simulink model "udp_signal"  (R2025b)
settings: Solver=VariableStepAuto  StartTime=0.0  StopTime=3600  RelTol=1e-3
undefined symbols (not defined in the file or in its folder): f
libraries: instrumentlib x2
settings Model: Creator=mateu  LastModifiedBy=mateu

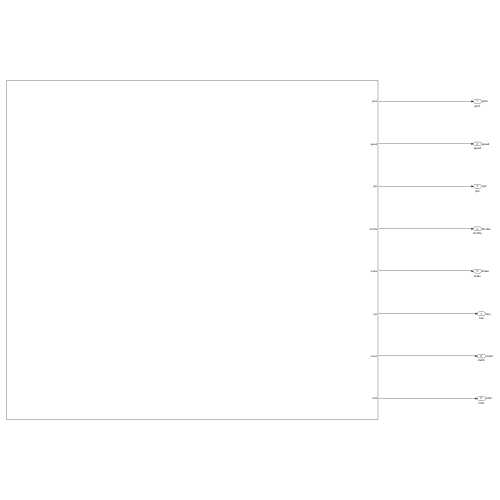
[thumbnail: Simulink's stored preview of the top-level diagram]
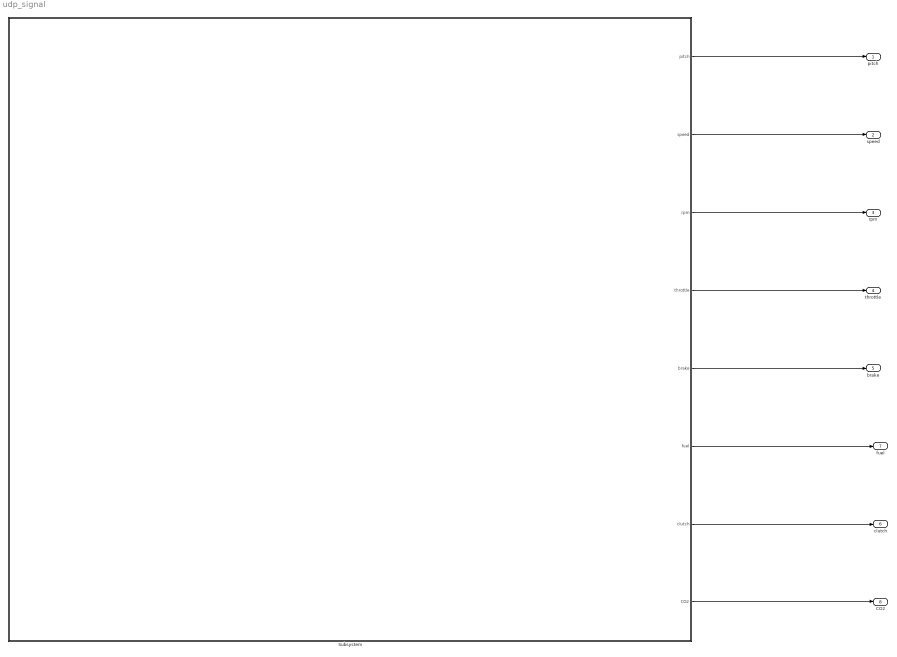
== system udp_signal ==
  Subsystem : Subsystem
  pitch : Outport  SignalName=pitch
  speed : Outport  Port=2  SignalName=speed
  rpm : Outport  Port=3  SignalName=rpm
  throttle : Outport  Port=4  SignalName=throttle
  brake : Outport  Port=5  SignalName=brake
  clutch : Outport  Port=6  SignalName=clutch
  fuel : Outport  Port=7  SignalName=fuel
  CO2 : Outport  Port=8  SignalName=CO2
  wires:
  Subsystem/1(pitch) -> pitch/1
  Subsystem/2(speed) -> speed/1
  Subsystem/3(rpm) -> rpm/1
  Subsystem/4(throttle) -> throttle/1
  Subsystem/5(brake) -> brake/1
  Subsystem/7(clutch) -> clutch/1
  Subsystem/6(fuel) -> fuel/1
  Subsystem/8(CO2) -> CO2/1

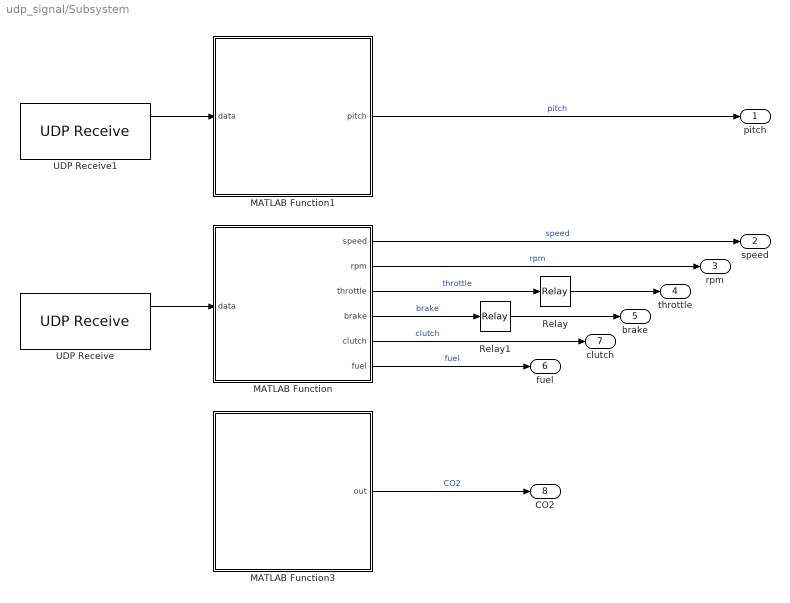
== system udp_signal/Subsystem ==
  MATLAB Function : MATLAB Function  TreatAsAtomicUnit=on
  MATLAB Function1 : MATLAB Function  TreatAsAtomicUnit=on
  MATLAB Function3 : MATLAB Function  TreatAsAtomicUnit=on  SystemSampleTime=0.001
  Relay : Relay  OnSwitchValue=0.75  OffSwitchValue=0.3
  Relay1 : Relay  OnSwitchValue=0.75  OffSwitchValue=0.3
  UDP Receive : instrumentlib/UDP Receive  LocalAddress=127.0.0.1  LocalPort=4444  EnablePortSharing=off  Host=localhost  Port=9090  GetLatestData=on  DataSize=[ 1, 96 ]  DataType=uint8  ASCIIFormatting=%f,  Terminator=LF  CustomTerminator=10  ByteOrder=big-endian  EnableBlockingMode=off  Timeout=10  SampleTime=0.01  SimulateUsing=Interpreted execution
  UDP Receive1 : instrumentlib/UDP Receive  LocalAddress=127.0.0.1  LocalPort=4445  EnablePortSharing=off  Host=localhost  Port=9090  GetLatestData=on  DataSize=[ 1, 88 ]  DataType=uint8  ASCIIFormatting=%f,  Terminator=LF  CustomTerminator=10  ByteOrder=big-endian  EnableBlockingMode=off  Timeout=10  SampleTime=0.01  SimulateUsing=Interpreted execution
  pitch : Outport
  speed : Outport  Port=2
  rpm : Outport  Port=3
  throttle : Outport  Port=4
  brake : Outport  Port=5
  fuel : Outport  Port=6
  clutch : Outport  Port=7
  CO2 : Outport  Port=8
  wires:
  MATLAB Function/4(brake) -> Relay1/1  "brake"
  MATLAB Function1/1(pitch) -> pitch/1  "pitch"
  UDP Receive1/1 -> MATLAB Function1/1(data)
  MATLAB Function/3(throttle) -> Relay/1  "throttle"
  MATLAB Function/1(speed) -> speed/1  "speed"
  MATLAB Function/2(rpm) -> rpm/1  "rpm"
  MATLAB Function3/1(out) -> CO2/1  "CO2"
  MATLAB Function/6(fuel) -> fuel/1  "fuel"
  UDP Receive/1 -> MATLAB Function/1(data)
  MATLAB Function/5(clutch) -> clutch/1  "clutch"
  Relay1/1 -> brake/1
  Relay/1 -> throttle/1

== matlab function udp_signal/Subsystem/MATLAB Function1 ==
  data: pitch output; data input
function pitch   = parse_pitch_beamng(data)
%#codegen

pitch    = single(0);

pitch = rad2deg(typecast(uint8(data(57:60)), 'single'));

== matlab function udp_signal/Subsystem/MATLAB Function ==
  data: speed output; rpm output; throttle output; brake output; clutch output; data input; fuel output
function [speed, rpm, throttle, brake, clutch, fuel ] = parse_beamng(data)
%#codegen

% =========================
% Force output types (IMPORTANT)
% =========================
speed    = single(0);
rpm      = single(0);
throttle = single(0);
brake    = single(0);
clutch   = single(0);
fuel     = single(0);

    
speed    = typecast(uint8(data(13:16)), 'single') * single(3.6);
rpm      = typecast(uint8(data(17:20)), 'single');
throttle = typecast(uint8(data(49:52)), 'single');
brake    = typecast(uint8(data(53:56)), 'single');
clutch   = typecast(uint8(data(57:60)), 'single');
fuel   = typecast(uint8(data(29:32)), 'single');

== matlab function udp_signal/Subsystem/MATLAB Function3 ==
  data: out output
function out = get_co2()

coder.extrinsic('get_co2_value');

out = single(0); % define output type

val = get_co2_value();

out = single(val);
